simulink model "controller"  (R2022a)
settings: Solver=ode5  StartTime=0.0  StopTime=10  FixedStep=Ts  MaxStep=Ts  RelTol=1e-3
model workspace (MAT data in the model file):
  Sig = Simulink.Signal
  Sig.DataType = 'auto'
  Sig.Dimensions = -1
  Sig.DimensionsMode = 'auto'
  Sig.Complexity = 'auto'
  Sig.SampleTime = -1
  Sig.SamplingMode = 'auto'
  Sig1 = Simulink.Signal
  Sig1.DataType = 'auto'
  Sig1.Dimensions = -1
  Sig1.DimensionsMode = 'auto'
  Sig1.Complexity = 'auto'
  Sig1.SampleTime = -1
  Sig1.SamplingMode = 'auto'
  Sig2 = Simulink.Signal
  Sig2.DataType = 'auto'
  Sig2.Dimensions = -1
  Sig2.DimensionsMode = 'auto'
  Sig2.Complexity = 'auto'
  Sig2.SampleTime = -1
  Sig2.SamplingMode = 'auto'
  Sig3 = Simulink.Signal
  Sig3.DataType = 'auto'
  Sig3.Dimensions = -1
  Sig3.DimensionsMode = 'auto'
  Sig3.Complexity = 'auto'
  Sig3.SampleTime = -1
  Sig3.SamplingMode = 'auto'
  Sig4 = Simulink.Signal
  Sig4.DataType = 'auto'
  Sig4.Dimensions = -1
  Sig4.DimensionsMode = 'auto'
  Sig4.Complexity = 'auto'
  Sig4.SampleTime = -1
  Sig4.SamplingMode = 'auto'
  Ts = 0.001
  benv = Simulink.Parameter
  benv.Value = 13.5
  benv.DataType = 'auto'
  benv.Complexity = 'real'
  benv.Dimensions = [1 1]
  bm = Simulink.Parameter
  bm.Value = 0.1
  bm.DataType = 'auto'
  bm.Complexity = 'real'
  bm.Dimensions = [1 1]
  bms = Simulink.Parameter
  bms.Value = 23.5
  bms.DataType = 'auto'
  bms.Complexity = 'real'
  bms.Dimensions = [1 1]
  bs = Simulink.Parameter
  bs.Value = 0.1
  bs.DataType = 'auto'
  bs.Complexity = 'real'
  bs.Dimensions = [1 1]
  ctrl_slct = Simulink.Parameter
  ctrl_slct.Value = 1
  ctrl_slct.DataType = 'auto'
  ctrl_slct.Complexity = 'real'
  ctrl_slct.Dimensions = [1 1]
  fm = Simulink.Parameter
  fm.Value = 1
  fm.DataType = 'auto'
  fm.Complexity = 'real'
  fm.Dimensions = [1 1]
  kenv = Simulink.Parameter
  kenv.Value = 50
  kenv.DataType = 'auto'
  kenv.Complexity = 'real'
  kenv.Dimensions = [1 1]
  kms = Simulink.Parameter
  kms.Value = 150
  kms.DataType = 'auto'
  kms.Complexity = 'real'
  kms.Dimensions = [1 1]
  mm = Simulink.Parameter
  mm.Value = 1
  mm.DataType = 'auto'
  mm.Complexity = 'real'
  mm.Dimensions = [1 1]
  mms = Simulink.Parameter
  mms.Value = 0.5
  mms.DataType = 'auto'
  mms.Complexity = 'real'
  mms.Dimensions = [1 1]
  ms = Simulink.Parameter
  ms.Value = 1
  ms.DataType = 'auto'
  ms.Complexity = 'real'
  ms.Dimensions = [1 1]
  um = Simulink.Parameter
  um.Value = 0.1
  um.DataType = 'auto'
  um.Complexity = 'real'
  um.Dimensions = [1 1]
  us = Simulink.Parameter
  us.Value = 0.1
  us.DataType = 'auto'
  us.Complexity = 'real'
  us.Dimensions = [1 1]
  xbar = Simulink.Parameter
  xbar.Value = 0.1
  xbar.DataType = 'auto'
  xbar.Complexity = 'real'
  xbar.Dimensions = [1 1]
settings Model: PauseTimes=1.3  Creator=jueda3  LastModifiedBy=xzhao
settings SolverCC: AlgebraicLoopSolver=TrustRegion  AutoInsertRateTranBlk=on
settings DataIOCC: LimitDataPoints=on  SaveFormat=Array  SignalLoggingSaveFormat=ModelDataLogs  ReturnWorkspaceOutputs=off  SignalLoggingName=sigsOut
settings OptimizationCC: DefaultParameterBehavior=Inlined  EnhancedBackFolding=on  PassReuseOutputArgsAs=Individual arguments  ZeroExternalMemoryAtStartup=off  ZeroInternalMemoryAtStartup=off  OptimizeBlockOrder=speed  DifferentSizesBufferReuse=on  OptimizationCustomize=off  EfficientTunableParamExpr=on
settings DebuggingCC: SaveWithParameterizedLinksMsg=none  UnderspecifiedInitializationDetection=Classic  MergeDetectMultiDrivingBlocksExec=none  SignalResolutionControl=TryResolveAllWithWarning  MultiTaskDSMMsg=warning  MultiTaskCondExecSysMsg=none  ParameterTunabilityLossMsg=error  UnconnectedInputMsg=warning  UnconnectedOutputMsg=warning  UnconnectedLineMsg=warning  SFMachineParentedDataDiag=warning  ArithmeticOperatorsInVariantConditions=warning
settings HardwareCC: ProdBitPerPointer=32  ProdBitPerSizeT=32  ProdBitPerPtrDiffT=32  ProdLargestAtomicFloat=None  ProdIntDivRoundTo=Undefined  ProdEndianess=Unspecified  ProdWordSize=32  ProdHWDeviceType=32-bit Generic  TargetBitPerPointer=64  TargetBitPerSizeT=64  TargetBitPerPtrDiffT=64  TargetLongLongMode=on  TargetIntDivRoundTo=Zero  TargetEndianess=LittleEndian  TargetWordSize=64  TargetHWDeviceType=MATLAB Host  ProdEqTarget=off
settings ModelReferenceCC: PropagateSignalLabelsOutOfModel=off
settings SFSimCC: SimUseLocalCustomCode=off  MATLABDynamicMemAlloc=off  CustomCodeUndefinedFunction=UseInterfaceOnly
settings RTWCC: Description=Embedded Coder (host-based shared library target)  SystemTargetFile=ert_shrlib.tlc  TemplateMakefile=ert_default_tmf  RTWUseLocalCustomCode=off  DLArmComputeVersion=19.05
settings CodeAppCC: ForceParamTrailComments=on  IgnoreCustomStorageClasses=off  OperatorAnnotations=on  SimulinkDataObjDesc=on  SFDataObjDesc=on  InsertBlockDesc=on
settings STFCustomTargetCC: MultiwordLength=256  GenerateSampleERTMain=on  ParMdlRefBuildCompliant=on  CompOptLevelCompliant=on  CombineOutputUpdateFcns=on  ERTCustomFileBanners=on  SupportContinuousTime=off  SupportNonInlinedSFcns=off  RemoveResetFunc=on  MATLABClassNameForMDSCustomization=Simulink.SoftwareTarget.ERTCustomization  ModelStepFunctionPrototypeControlCompliant=on  GRTInterface=off  UseToolchainInfoCompliant=on  SystemTargetFile=ert_shrlib.tlc
settings ERTTargetCC: GenerateSampleERTMain=on  ConcurrentExecutionCompliant=off  CPPClassGenCompliant=off  InlinedParameterPlacement=NonHierarchical  ERTCustomFileTemplate=example_file_process.tlc
settings ConfigComp: CovMetricSettings=dw  CovSaveCumulativeToWorkspaceVar=on  CovSaveSingleToWorkspaceVar=on  CovExternalEMLEnable=off

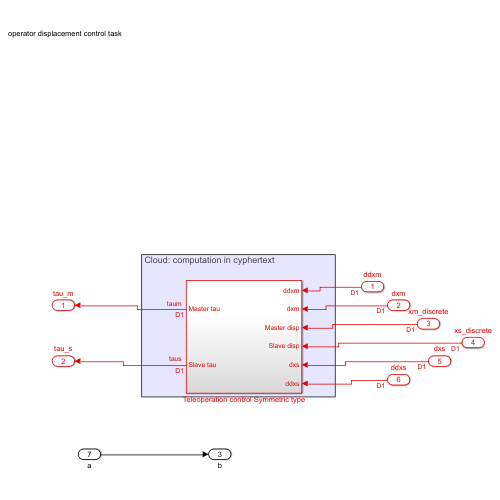
[thumbnail: Simulink's stored preview of the top-level diagram]
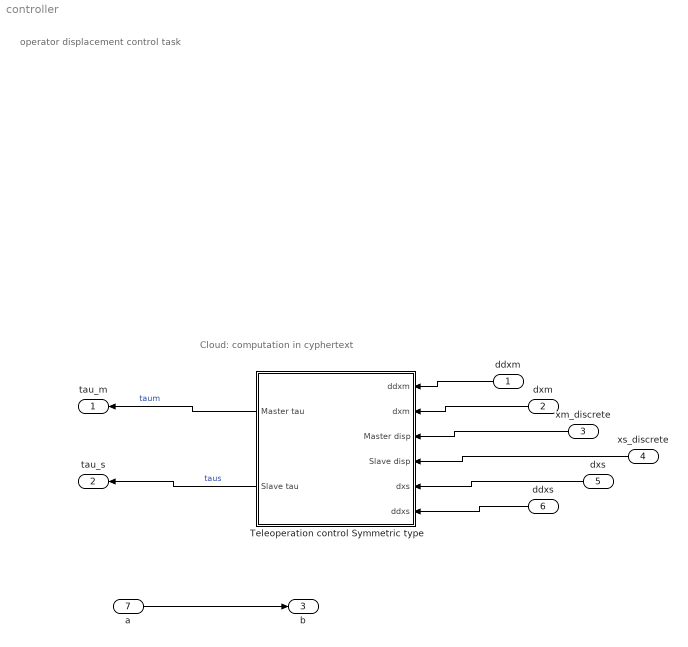
== system controller ==
  note: Cloud: computation in cyphertext
  note: operator displacement control task
  ddxm : Inport
  dxm : Inport  Port=2
  xm_discrete : Inport  Port=3
  xs_discrete : Inport  Port=4
  dxs : Inport  Port=5
  ddxs : Inport  Port=6
  a : Inport  Port=7
  Teleoperation control Symmetric type : Subsystem
  tau_m : Outport
  tau_s : Outport  Port=2
  b : Outport  Port=3
  wires:
  Teleoperation control Symmetric type/1(Master tau) -> tau_m/1  "taum"
  Teleoperation control Symmetric type/2(Slave tau) -> tau_s/1  "taus"
  ddxm/1 -> Teleoperation control Symmetric type/1(ddxm)
  dxm/1 -> Teleoperation control Symmetric type/2(dxm)
  xm_discrete/1 -> Teleoperation control Symmetric type/3(Master disp)
  xs_discrete/1 -> Teleoperation control Symmetric type/4(Slave disp)
  dxs/1 -> Teleoperation control Symmetric type/5(dxs)
  ddxs/1 -> Teleoperation control Symmetric type/6(ddxs)
  a/1 -> b/1

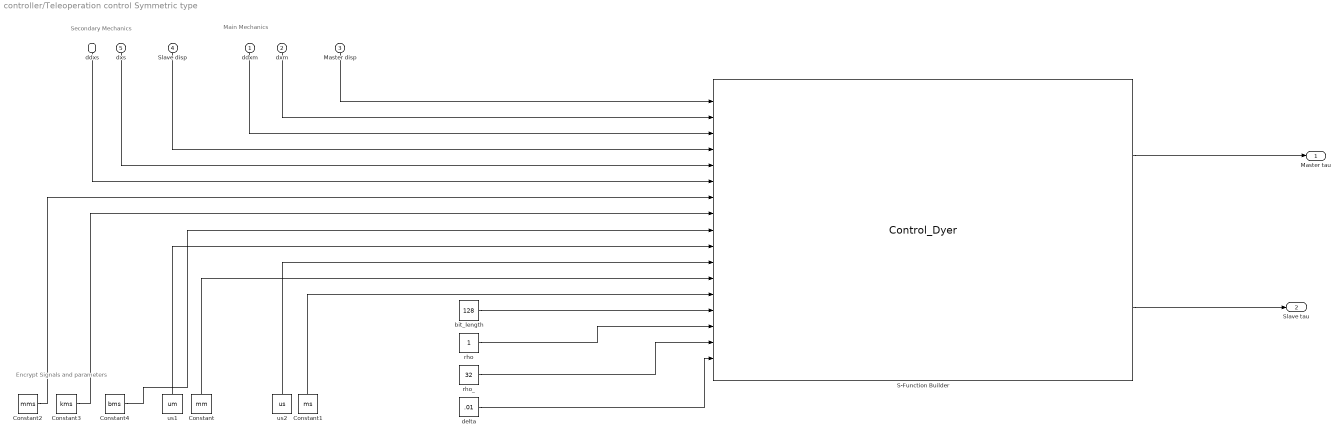
== system controller/Teleoperation control Symmetric type ==
  note: Encrypt Signals and parameters
  note: Secondary Mechanics
  note: Main Mechanics
  ddxm : Inport
  dxm : Inport  Port=2
  Master disp : Inport  Port=3
  Slave disp : Inport  Port=4
  dxs : Inport  Port=5
  ddxs : Inport  Port=6
  Constant : Constant  Value=mm
  Constant1 : Constant  Value=ms
  Constant2 : Constant  Value=mms
  Constant3 : Constant  Value=kms
  Constant4 : Constant  Value=bms
  S-Function Builder : S-Function  FunctionName=Control_Dyer  Parameters=1  SFunctionModules=Control_Dyer_wrapper  SFunctionDeploymentMode=off  EnableBusSupport=off  mask(S-Function Builder){}
      mask help: Simulink:masks:SFunctionBuilder_MD
      mask init:
      | val = [[.9  0.75 0.75 1 1 .9 .9 1]',[1 1 0.75 0.75 .9 .9 1 .9]'];try , sys = get_param(gcb,'SfunBuilderFcnName');if isempty(sys), sys = get_param(gcb,'FunctionName'); end,catch, sys = get_param(gcb,'FunctionName'); end
      settings: CopyFcn=set_param(gcbh,'LinkStatus','none')  OpenFcn=sfunctionwizard(gcbh)
      mask Display:
      | plot(val(:,1),val(:,2))
      | disp(sys)
      | port_label('input',1,'xm')
      | port_label('input',2,'dxm')
      | port_label('input',3,'ddxm')
      | port_label('input',4,'xs')
      | port_label('input',5,'dxs')
      | port_label('input',6,'ddxs')
      | port_label('input',7,'mms')
      | port_label('input',8,'kms')
      | port_label('input',9,'bms')
      | port_label('input',10,'um')
      | port_label('input',11,'us')
      | port_label('input',12,'mm')
      | port_label('input',13,'ms')
      | port_label('input',14,'bit_length')
      | port_label('input',15,'rho')
      | port_label('input',16,'rho_')
      | port_label('input',17,'delta')
      | port_label('output',1,'tau_m')
      | port_label('output',2,'tau_s')
  bit_length : Constant  Value=128
  delta : Constant  Value=.01
  rho : Constant
  rho_ : Constant  Value=32
  us1 : Constant  Value=um
  us2 : Constant  Value=us
  Master tau : Outport
  Slave tau : Outport  Port=2
  wires:
  Master disp/1 -> S-Function Builder/1
  Slave disp/1 -> S-Function Builder/4
  Constant2/1 -> S-Function Builder/7
  Constant3/1 -> S-Function Builder/8
  Constant4/1 -> S-Function Builder/9
  us1/1 -> S-Function Builder/10
  us2/1 -> S-Function Builder/11
  Constant/1 -> S-Function Builder/12
  Constant1/1 -> S-Function Builder/13
  dxm/1 -> S-Function Builder/2
  ddxm/1 -> S-Function Builder/3
  dxs/1 -> S-Function Builder/5
  ddxs/1 -> S-Function Builder/6
  S-Function Builder/1 -> Master tau/1
  S-Function Builder/2 -> Slave tau/1
  bit_length/1 -> S-Function Builder/14
  rho/1 -> S-Function Builder/15
  rho_/1 -> S-Function Builder/16
  delta/1 -> S-Function Builder/17
